simulink model "AM_Multiple_Channels"  (R2014b)
settings: Solver=ode3  StartTime=0.0  StopTime=6  FixedStep=1/5000000  RelTol=1e-3
undefined symbols (not defined in the file or in its folder): dfilt, fdesignblkfcn, gcbh
libraries: dsparch4 x12, commsynccomp2 x8, simulink x8
settings Model: Creator=Eitima  LastModifiedBy=Eitima
settings DataIOCC: ExternalInput=[t,SigTime]  LimitDataPoints=off  LoadExternalInput=on  TimeSaveName=tOut  OutputSaveName=SigTimeOut

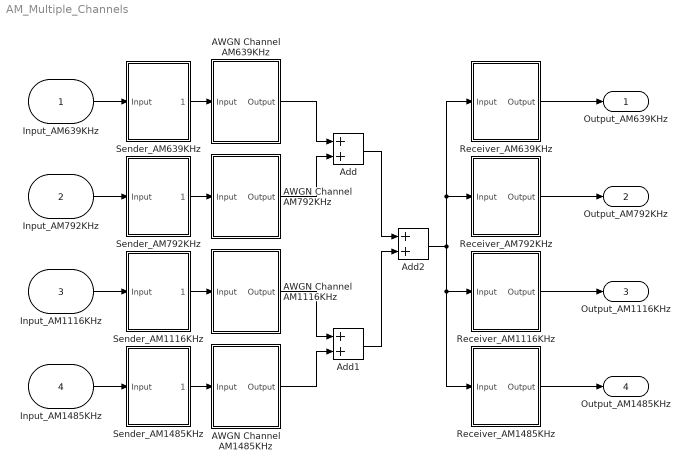
== system AM_Multiple_Channels ==
  Input_AM639KHz : Inport
  Input_AM792KHz : Inport  Port=2
  Input_AM1116KHz : Inport  Port=3
  Input_AM1485KHz : Inport  Port=4
  AWGN Channel AM1116KHz : Subsystem
  AWGN Channel AM1485KHz : Subsystem
  AWGN Channel AM639KHz : Subsystem
  AWGN Channel AM792KHz : Subsystem
  Add : Sum
  Add1 : Sum
  Add2 : Sum
  Receiver_AM1116KHz : Subsystem
  Receiver_AM1485KHz : Subsystem
  Receiver_AM639KHz : Subsystem
  Receiver_AM792KHz : Subsystem
  Sender_AM1116KHz : Subsystem
  Sender_AM1485KHz : Subsystem
  "Sender_AM639KHz " : Subsystem
  Sender_AM792KHz : Subsystem
  Output_AM639KHz : Outport
  Output_AM792KHz : Outport  Port=2
  Output_AM1116KHz : Outport  Port=3
  Output_AM1485KHz : Outport  Port=4
  wires:
  Input_AM639KHz/1 -> "Sender_AM639KHz "/1(Input)
  "Sender_AM639KHz "/1(Output) -> AWGN Channel AM639KHz/1(Input)
  AWGN Channel AM639KHz/1(Output) -> Add/1
  Input_AM792KHz/1 -> Sender_AM792KHz/1(Input)
  Input_AM1116KHz/1 -> Sender_AM1116KHz/1(Input)
  Input_AM1485KHz/1 -> Sender_AM1485KHz/1(Input)
  Sender_AM792KHz/1(Output) -> AWGN Channel AM792KHz/1(Input)
  AWGN Channel AM792KHz/1(Output) -> Add/2
  Sender_AM1116KHz/1(Output) -> AWGN Channel AM1116KHz/1(Input)
  Sender_AM1485KHz/1(Output) -> AWGN Channel AM1485KHz/1(Input)
  AWGN Channel AM1116KHz/1(Output) -> Add1/1
  AWGN Channel AM1485KHz/1(Output) -> Add1/2
  Receiver_AM639KHz/1(Output) -> Output_AM639KHz/1
  Add2/1 -> Receiver_AM1485KHz/1(Input), Receiver_AM1116KHz/1(Input), Receiver_AM792KHz/1(Input), Receiver_AM639KHz/1(Input)
  Add/1 -> Add2/1
  Add1/1 -> Add2/2
  Receiver_AM792KHz/1(Output) -> Output_AM792KHz/1
  Receiver_AM1116KHz/1(Output) -> Output_AM1116KHz/1
  Receiver_AM1485KHz/1(Output) -> Output_AM1485KHz/1

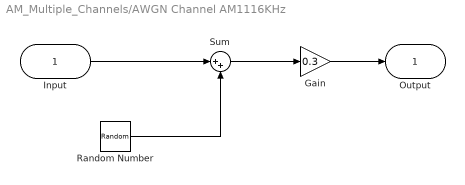
== system AM_Multiple_Channels/AWGN Channel AM1116KHz ==
  Input : Inport
  Gain : Gain  Gain=0.3
  Random Number : RandomNumber  Variance=0.01  Seed=69  SampleTime=1/5000000
  Sum : Sum  Inputs=|++
  Output : Outport
  wires:
  Random Number/1 -> Sum/2
  Input/1 -> Sum/1
  Sum/1 -> Gain/1
  Gain/1 -> Output/1

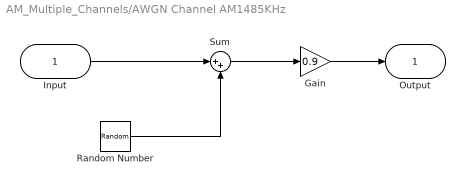
== system AM_Multiple_Channels/AWGN Channel AM1485KHz ==
  Input : Inport
  Gain : Gain  Gain=0.9
  Random Number : RandomNumber  Variance=0.01  Seed=70  SampleTime=1/5000000
  Sum : Sum  Inputs=|++
  Output : Outport
  wires:
  Random Number/1 -> Sum/2
  Input/1 -> Sum/1
  Sum/1 -> Gain/1
  Gain/1 -> Output/1

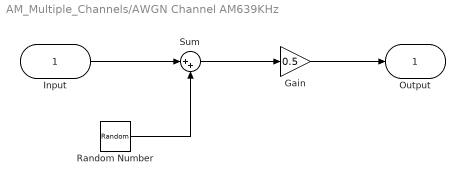
== system AM_Multiple_Channels/AWGN Channel AM639KHz ==
  Input : Inport
  Gain : Gain  Gain=0.5
  Random Number : RandomNumber  Variance=0.01  Seed=64  SampleTime=1/5000000
  Sum : Sum  Inputs=|++
  Output : Outport
  wires:
  Random Number/1 -> Sum/2
  Input/1 -> Sum/1
  Sum/1 -> Gain/1
  Gain/1 -> Output/1

== system AM_Multiple_Channels/AWGN Channel AM792KHz ==
  Input : Inport
  Gain : Gain
  Random Number : RandomNumber  Variance=0.01  Seed=67  SampleTime=1/5000000
  Sum : Sum  Inputs=|++
  Output : Outport
  wires:
  Random Number/1 -> Sum/2
  Input/1 -> Sum/1
  Sum/1 -> Gain/1
  Gain/1 -> Output/1

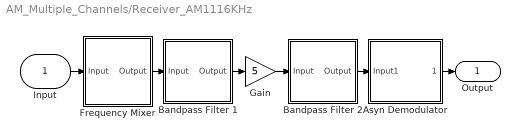
== system AM_Multiple_Channels/Receiver_AM1116KHz ==
  Input : Inport
  Asyn Demodulator : Subsystem
  Bandpass Filter 1 : Subsystem
  Bandpass Filter 2 : Subsystem
  "Frequency Mixer " : Subsystem
  Gain : Gain  Gain=5
  Output : Outport
  wires:
  Input/1 -> "Frequency Mixer "/1(Input)
  "Frequency Mixer "/1(Output) -> Bandpass Filter 1/1(Input)
  Bandpass Filter 1/1(Output) -> Gain/1
  Gain/1 -> Bandpass Filter 2/1(Input)
  Bandpass Filter 2/1(Output) -> Asyn Demodulator/1(Input1)
  Asyn Demodulator/1(Output1) -> Output/1

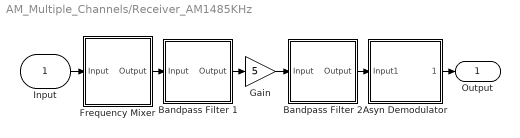
== system AM_Multiple_Channels/Receiver_AM1485KHz ==
  Input : Inport
  Asyn Demodulator : Subsystem
  Bandpass Filter 1 : Subsystem
  Bandpass Filter 2 : Subsystem
  "Frequency Mixer " : Subsystem
  Gain : Gain  Gain=5
  Output : Outport
  wires:
  Input/1 -> "Frequency Mixer "/1(Input)
  "Frequency Mixer "/1(Output) -> Bandpass Filter 1/1(Input)
  Bandpass Filter 1/1(Output) -> Gain/1
  Gain/1 -> Bandpass Filter 2/1(Input)
  Bandpass Filter 2/1(Output) -> Asyn Demodulator/1(Input1)
  Asyn Demodulator/1(Output1) -> Output/1

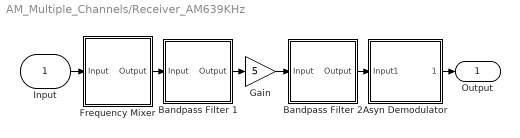
== system AM_Multiple_Channels/Receiver_AM639KHz ==
  Input : Inport
  Asyn Demodulator : Subsystem
  Bandpass Filter 1 : Subsystem
  Bandpass Filter 2 : Subsystem
  "Frequency Mixer " : Subsystem
  Gain : Gain  Gain=5
  Output : Outport
  wires:
  Input/1 -> "Frequency Mixer "/1(Input)
  "Frequency Mixer "/1(Output) -> Bandpass Filter 1/1(Input)
  Bandpass Filter 1/1(Output) -> Gain/1
  Gain/1 -> Bandpass Filter 2/1(Input)
  Bandpass Filter 2/1(Output) -> Asyn Demodulator/1(Input1)
  Asyn Demodulator/1(Output1) -> Output/1

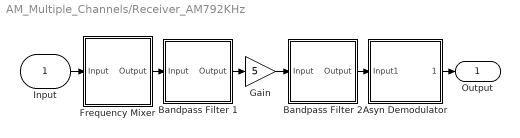
== system AM_Multiple_Channels/Receiver_AM792KHz ==
  Input : Inport
  Asyn Demodulator : Subsystem
  Bandpass Filter 1 : Subsystem
  Bandpass Filter 2 : Subsystem
  "Frequency Mixer " : Subsystem
  Gain : Gain  Gain=5
  Output : Outport
  wires:
  Input/1 -> "Frequency Mixer "/1(Input)
  "Frequency Mixer "/1(Output) -> Bandpass Filter 1/1(Input)
  Bandpass Filter 1/1(Output) -> Gain/1
  Gain/1 -> Bandpass Filter 2/1(Input)
  Bandpass Filter 2/1(Output) -> Asyn Demodulator/1(Input1)
  Asyn Demodulator/1(Output1) -> Output/1

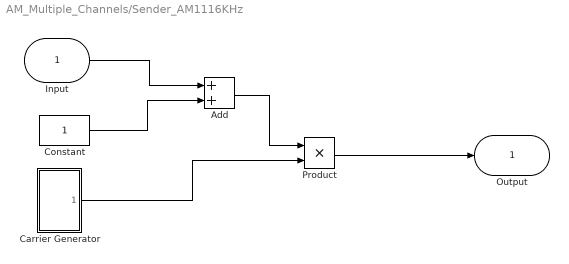
== system AM_Multiple_Channels/Sender_AM1116KHz ==
  Input : Inport
  Add : Sum
  Carrier Generator : Subsystem
  Constant : Constant
  Product : Product
  Output : Outport
  wires:
  Input/1 -> Add/1
  Constant/1 -> Add/2
  Product/1 -> Output/1
  Add/1 -> Product/1
  Carrier Generator/1(Carrier) -> Product/2

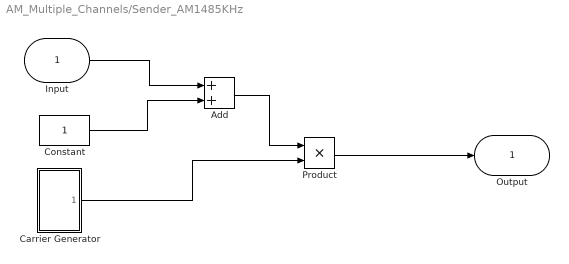
== system AM_Multiple_Channels/Sender_AM1485KHz ==
  Input : Inport
  Add : Sum
  Carrier Generator : Subsystem
  Constant : Constant
  Product : Product
  Output : Outport
  wires:
  Input/1 -> Add/1
  Constant/1 -> Add/2
  Product/1 -> Output/1
  Add/1 -> Product/1
  Carrier Generator/1(Carrier) -> Product/2

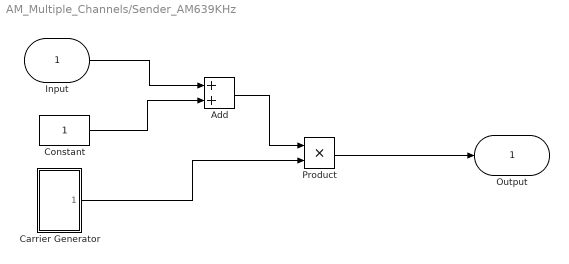
== system AM_Multiple_Channels/Sender_AM639KHz  ==
  Input : Inport
  Add : Sum
  Carrier Generator : Subsystem
  Constant : Constant
  Product : Product
  Output : Outport
  wires:
  Input/1 -> Add/1
  Constant/1 -> Add/2
  Product/1 -> Output/1
  Add/1 -> Product/1
  Carrier Generator/1(Carrier) -> Product/2

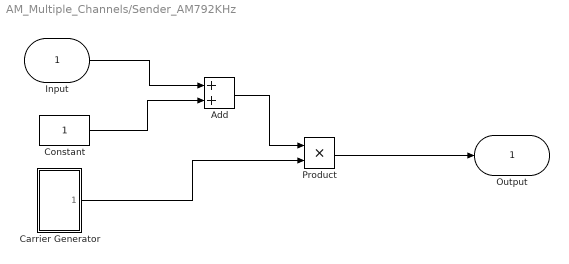
== system AM_Multiple_Channels/Sender_AM792KHz ==
  Input : Inport
  Add : Sum
  Carrier Generator : Subsystem
  Constant : Constant
  Product : Product
  Output : Outport
  wires:
  Input/1 -> Add/1
  Constant/1 -> Add/2
  Product/1 -> Output/1
  Add/1 -> Product/1
  Carrier Generator/1(Carrier) -> Product/2

== system AM_Multiple_Channels/Receiver_AM1116KHz/Asyn Demodulator ==
  Input1 : Inport
  Lowpass Filter1 : Subsystem
  Saturation : Saturate  UpperLimit=inf  LowerLimit=0
  Output1 : Outport
  wires:
  Lowpass Filter1/1(Output) -> Output1/1
  Saturation/1 -> Lowpass Filter1/1(Input)
  Input1/1 -> Saturation/1

== system AM_Multiple_Channels/Receiver_AM1116KHz/Bandpass Filter 1 ==
  Input : Inport
  Bandpass Filter1 : Subsystem  DialogController=fdesignblkfcn  InitFcn=fdesignblkfcn(gcbh, {'InitFcn'});  mask(Bandpass Filter){}
      mask help: Design a bandpass filter
      settings: CopyFcn=fdesignblkfcn(gcbh, {'CopyFcn'});
      mask Help: helpview(mapfilelocation('dsp'), 'dspbandpassfilter');
      mask Display: disp('Bandpass');
  Reshape1 : Reshape
  Zero-Order Hold : ZeroOrderHold  SampleTime=-1
  Output : Outport
  wires:
  Zero-Order Hold/1 -> Bandpass Filter1/1(In)
  Input/1 -> Zero-Order Hold/1
  Bandpass Filter1/1(Out) -> Reshape1/1
  Reshape1/1 -> Output/1

== system AM_Multiple_Channels/Receiver_AM1116KHz/Bandpass Filter 2 ==
  Input : Inport
  Bandpass Filter1 : Subsystem  DialogController=fdesignblkfcn  InitFcn=fdesignblkfcn(gcbh, {'InitFcn'});  mask(Bandpass Filter){}
      mask help: Design a bandpass filter
      settings: CopyFcn=fdesignblkfcn(gcbh, {'CopyFcn'});
      mask Help: helpview(mapfilelocation('dsp'), 'dspbandpassfilter');
      mask Display: disp('Bandpass');
  Reshape1 : Reshape
  Zero-Order Hold1 : ZeroOrderHold  SampleTime=-1
  Output : Outport
  wires:
  Zero-Order Hold1/1 -> Bandpass Filter1/1(In)
  Input/1 -> Zero-Order Hold1/1
  Bandpass Filter1/1(Out) -> Reshape1/1
  Reshape1/1 -> Output/1

== system AM_Multiple_Channels/Receiver_AM1116KHz/Frequency Mixer  ==
  Input : Inport
  Local Oscilator Signal : Subsystem
  Product : Product
  Output : Outport
  wires:
  Product/1 -> Output/1
  Local Oscilator Signal/1(Output) -> Product/2
  Input/1 -> Product/1

== system AM_Multiple_Channels/Receiver_AM1485KHz/Asyn Demodulator ==
  Input1 : Inport
  Lowpass Filter1 : Subsystem
  Saturation : Saturate  UpperLimit=inf  LowerLimit=0
  Output1 : Outport
  wires:
  Lowpass Filter1/1(Output) -> Output1/1
  Saturation/1 -> Lowpass Filter1/1(Input)
  Input1/1 -> Saturation/1

== system AM_Multiple_Channels/Receiver_AM1485KHz/Bandpass Filter 1 ==
  Input : Inport
  Bandpass Filter1 : Subsystem  DialogController=fdesignblkfcn  InitFcn=fdesignblkfcn(gcbh, {'InitFcn'});  mask(Bandpass Filter){}
      mask help: Design a bandpass filter
      settings: CopyFcn=fdesignblkfcn(gcbh, {'CopyFcn'});
      mask Help: helpview(mapfilelocation('dsp'), 'dspbandpassfilter');
      mask Display: disp('Bandpass');
  Reshape1 : Reshape
  Zero-Order Hold : ZeroOrderHold  SampleTime=-1
  Output : Outport
  wires:
  Zero-Order Hold/1 -> Bandpass Filter1/1(In)
  Input/1 -> Zero-Order Hold/1
  Bandpass Filter1/1(Out) -> Reshape1/1
  Reshape1/1 -> Output/1

== system AM_Multiple_Channels/Receiver_AM1485KHz/Bandpass Filter 2 ==
  Input : Inport
  Bandpass Filter1 : Subsystem  DialogController=fdesignblkfcn  InitFcn=fdesignblkfcn(gcbh, {'InitFcn'});  mask(Bandpass Filter){}
      mask help: Design a bandpass filter
      settings: CopyFcn=fdesignblkfcn(gcbh, {'CopyFcn'});
      mask Help: helpview(mapfilelocation('dsp'), 'dspbandpassfilter');
      mask Display: disp('Bandpass');
  Reshape1 : Reshape
  Zero-Order Hold1 : ZeroOrderHold  SampleTime=-1
  Output : Outport
  wires:
  Zero-Order Hold1/1 -> Bandpass Filter1/1(In)
  Input/1 -> Zero-Order Hold1/1
  Bandpass Filter1/1(Out) -> Reshape1/1
  Reshape1/1 -> Output/1

== system AM_Multiple_Channels/Receiver_AM1485KHz/Frequency Mixer  ==
  Input : Inport
  Local Oscilator Signal : Subsystem
  Product : Product
  Output : Outport
  wires:
  Product/1 -> Output/1
  Local Oscilator Signal/1(Output) -> Product/2
  Input/1 -> Product/1

== system AM_Multiple_Channels/Receiver_AM639KHz/Asyn Demodulator ==
  Input1 : Inport
  Lowpass Filter1 : Subsystem
  Saturation : Saturate  UpperLimit=inf  LowerLimit=0
  Output1 : Outport
  wires:
  Lowpass Filter1/1(Output) -> Output1/1
  Saturation/1 -> Lowpass Filter1/1(Input)
  Input1/1 -> Saturation/1

== system AM_Multiple_Channels/Receiver_AM639KHz/Bandpass Filter 1 ==
  Input : Inport
  Bandpass Filter1 : Subsystem  DialogController=fdesignblkfcn  InitFcn=fdesignblkfcn(gcbh, {'InitFcn'});  mask(Bandpass Filter){}
      mask help: Design a bandpass filter
      settings: CopyFcn=fdesignblkfcn(gcbh, {'CopyFcn'});
      mask Help: helpview(mapfilelocation('dsp'), 'dspbandpassfilter');
      mask Display: disp('Bandpass');
  Reshape1 : Reshape
  Zero-Order Hold : ZeroOrderHold  SampleTime=-1
  Output : Outport
  wires:
  Zero-Order Hold/1 -> Bandpass Filter1/1(In)
  Input/1 -> Zero-Order Hold/1
  Bandpass Filter1/1(Out) -> Reshape1/1
  Reshape1/1 -> Output/1

== system AM_Multiple_Channels/Receiver_AM639KHz/Bandpass Filter 2 ==
  Input : Inport
  Bandpass Filter1 : Subsystem  DialogController=fdesignblkfcn  InitFcn=fdesignblkfcn(gcbh, {'InitFcn'});  mask(Bandpass Filter){}
      mask help: Design a bandpass filter
      settings: CopyFcn=fdesignblkfcn(gcbh, {'CopyFcn'});
      mask Help: helpview(mapfilelocation('dsp'), 'dspbandpassfilter');
      mask Display: disp('Bandpass');
  Reshape1 : Reshape
  Zero-Order Hold1 : ZeroOrderHold  SampleTime=-1
  Output : Outport
  wires:
  Zero-Order Hold1/1 -> Bandpass Filter1/1(In)
  Input/1 -> Zero-Order Hold1/1
  Bandpass Filter1/1(Out) -> Reshape1/1
  Reshape1/1 -> Output/1

== system AM_Multiple_Channels/Receiver_AM639KHz/Frequency Mixer  ==
  Input : Inport
  Local Oscilator Signal : Subsystem
  Product : Product
  Output : Outport
  wires:
  Product/1 -> Output/1
  Local Oscilator Signal/1(Output) -> Product/2
  Input/1 -> Product/1

== system AM_Multiple_Channels/Receiver_AM792KHz/Asyn Demodulator ==
  Input1 : Inport
  Lowpass Filter1 : Subsystem
  Saturation : Saturate  UpperLimit=inf  LowerLimit=0
  Output1 : Outport
  wires:
  Lowpass Filter1/1(Output) -> Output1/1
  Saturation/1 -> Lowpass Filter1/1(Input)
  Input1/1 -> Saturation/1

== system AM_Multiple_Channels/Receiver_AM792KHz/Bandpass Filter 1 ==
  Input : Inport
  Bandpass Filter1 : Subsystem  DialogController=fdesignblkfcn  InitFcn=fdesignblkfcn(gcbh, {'InitFcn'});  mask(Bandpass Filter){}
      mask help: Design a bandpass filter
      settings: CopyFcn=fdesignblkfcn(gcbh, {'CopyFcn'});
      mask Help: helpview(mapfilelocation('dsp'), 'dspbandpassfilter');
      mask Display: disp('Bandpass');
  Reshape1 : Reshape
  Zero-Order Hold : ZeroOrderHold  SampleTime=-1
  Output : Outport
  wires:
  Zero-Order Hold/1 -> Bandpass Filter1/1(In)
  Input/1 -> Zero-Order Hold/1
  Bandpass Filter1/1(Out) -> Reshape1/1
  Reshape1/1 -> Output/1

== system AM_Multiple_Channels/Receiver_AM792KHz/Bandpass Filter 2 ==
  Input : Inport
  Bandpass Filter1 : Subsystem  DialogController=fdesignblkfcn  InitFcn=fdesignblkfcn(gcbh, {'InitFcn'});  mask(Bandpass Filter){}
      mask help: Design a bandpass filter
      settings: CopyFcn=fdesignblkfcn(gcbh, {'CopyFcn'});
      mask Help: helpview(mapfilelocation('dsp'), 'dspbandpassfilter');
      mask Display: disp('Bandpass');
  Reshape1 : Reshape
  Zero-Order Hold1 : ZeroOrderHold  SampleTime=-1
  Output : Outport
  wires:
  Zero-Order Hold1/1 -> Bandpass Filter1/1(In)
  Input/1 -> Zero-Order Hold1/1
  Bandpass Filter1/1(Out) -> Reshape1/1
  Reshape1/1 -> Output/1

== system AM_Multiple_Channels/Receiver_AM792KHz/Frequency Mixer  ==
  Input : Inport
  Local Oscilator Signal : Subsystem
  Product : Product
  Output : Outport
  wires:
  Product/1 -> Output/1
  Local Oscilator Signal/1(Output) -> Product/2
  Input/1 -> Product/1

== system AM_Multiple_Channels/Sender_AM1116KHz/Carrier Generator ==
  Constant1 : Constant
  Discrete-Time VCO : commsynccomp2/Discrete-Time VCO  Ac=1  Fc=0  Kc=1000  Ph=0  ts=1/5000000
  Slider Gain : simulink/Math Operations/Slider Gain  low=550  gain=1116  high=1605
  Carrier : Outport
  wires:
  Discrete-Time VCO/1 -> Carrier/1
  Slider Gain/1 -> Discrete-Time VCO/1
  Constant1/1 -> Slider Gain/1

== system AM_Multiple_Channels/Sender_AM1485KHz/Carrier Generator ==
  Constant1 : Constant
  Discrete-Time VCO : commsynccomp2/Discrete-Time VCO  Ac=1  Fc=0  Kc=1000  Ph=0  ts=1/5000000
  Slider Gain : simulink/Math Operations/Slider Gain  low=550  gain=1485  high=1605
  Carrier : Outport
  wires:
  Discrete-Time VCO/1 -> Carrier/1
  Slider Gain/1 -> Discrete-Time VCO/1
  Constant1/1 -> Slider Gain/1

== system AM_Multiple_Channels/Sender_AM639KHz /Carrier Generator ==
  Constant1 : Constant
  Discrete-Time VCO : commsynccomp2/Discrete-Time VCO  Ac=1  Fc=0  Kc=1000  Ph=0  ts=1/5000000
  Slider Gain : simulink/Math Operations/Slider Gain  low=550  gain=639  high=1605
  Carrier : Outport
  wires:
  Discrete-Time VCO/1 -> Carrier/1
  Slider Gain/1 -> Discrete-Time VCO/1
  Constant1/1 -> Slider Gain/1

== system AM_Multiple_Channels/Sender_AM792KHz/Carrier Generator ==
  Constant1 : Constant
  Discrete-Time VCO : commsynccomp2/Discrete-Time VCO  Ac=1  Fc=0  Kc=1000  Ph=0  ts=1/5000000
  Slider Gain : simulink/Math Operations/Slider Gain  low=550  gain=792  high=1605
  Carrier : Outport
  wires:
  Discrete-Time VCO/1 -> Carrier/1
  Slider Gain/1 -> Discrete-Time VCO/1
  Constant1/1 -> Slider Gain/1

== system AM_Multiple_Channels/Receiver_AM1116KHz/Asyn Demodulator/Lowpass Filter1 ==
  Input : Inport
  Lowpass Filter : Subsystem  DialogController=fdesignblkfcn  InitFcn=fdesignblkfcn(gcbh, {'InitFcn'});  mask(Lowpass Filter){}
      mask help: Design a lowpass filter
      settings: CopyFcn=fdesignblkfcn(gcbh, {'CopyFcn'});
      mask Help: helpview(mapfilelocation('dsp'), 'dsplowpassfilter');
      mask Display: disp('Lowpass')
  Reshape : Reshape
  Zero-Order Hold1 : ZeroOrderHold  SampleTime=-1
  Output : Outport
  wires:
  Zero-Order Hold1/1 -> Lowpass Filter/1(In)
  Input/1 -> Zero-Order Hold1/1
  Lowpass Filter/1(Out) -> Reshape/1
  Reshape/1 -> Output/1

== system AM_Multiple_Channels/Receiver_AM1116KHz/Bandpass Filter 1/Bandpass Filter1 ==
  In : Inport
  Generated Filter Block : dsparch4/Biquad Filter  Tag=BlockMethodSubSystem  IIRFiltStruct=Direct form II  CoeffSource=Specify via dialog  BiQuadCoeffs=[0.01013958648634297 0 -0.01013958648634297 1 -1.6618133812024951 0.98627046054740486;0.0025493781187891492 0 -0.0025493781187891492 1 -1.6514591991218408 0.98607730419032968;0.016304485317952876 0 -0.016304485317952876 1 -1.6744504392878072 0.99677925049276372;0.010019474414157988 0 -0.010019474414157988 1 -1.6562936076737262 0.99669840495107032;0.011567698875754661 0 -0.011567698875754661 1 -1.6564338939134684 0.98375080085450683;0.0047790385123797378 0 -0.0047790385123797378 1 -1.6527923586273903 0.98367098468879577;0.014421092390225715 0 -0.014421092390225715 1 -1.6681267322604891 0.99083770350510236;0.91340939446196634 0 -0.91340939446196634 1 -1.6526752268318703 0.99064368018868598]  a0Flag=Warning  IC=0  ICnum=0  ICden=0  InputProcessing=Columns as channels (frame based)  denAccumFracLength=30  denProdOutputFracLength=30  secondMemoryFracLength=15  roundingMode=Floor  overflowMode=off  ScaleValues=[0.0075209697231768506;1;1;1;1;1;1;1;1]  optimizeScaleValues=off  ScaleValueMode=Specify via input port (g)  scaleValueFracLength=14  FilterSource=Specify via dialog  dfiltObjectName=dfilt.df2tsos([1 0.3 0.4],[1 0.1 0.2])
  Out : Outport
  wires:
  Generated Filter Block/1 -> Out/1
  In/1 -> Generated Filter Block/1

== system AM_Multiple_Channels/Receiver_AM1116KHz/Bandpass Filter 2/Bandpass Filter1 ==
  In : Inport
  Generated Filter Block : dsparch4/Biquad Filter  Tag=BlockMethodSubSystem  IIRFiltStruct=Direct form II  CoeffSource=Specify via dialog  BiQuadCoeffs=[0.01013958648634297 0 -0.01013958648634297 1 -1.6618133812024951 0.98627046054740486;0.0025493781187891492 0 -0.0025493781187891492 1 -1.6514591991218408 0.98607730419032968;0.016304485317952876 0 -0.016304485317952876 1 -1.6744504392878072 0.99677925049276372;0.010019474414157988 0 -0.010019474414157988 1 -1.6562936076737262 0.99669840495107032;0.011567698875754661 0 -0.011567698875754661 1 -1.6564338939134684 0.98375080085450683;0.0047790385123797378 0 -0.0047790385123797378 1 -1.6527923586273903 0.98367098468879577;0.014421092390225715 0 -0.014421092390225715 1 -1.6681267322604891 0.99083770350510236;0.91340939446196634 0 -0.91340939446196634 1 -1.6526752268318703 0.99064368018868598]  a0Flag=Warning  IC=0  ICnum=0  ICden=0  InputProcessing=Columns as channels (frame based)  denAccumFracLength=30  denProdOutputFracLength=30  secondMemoryFracLength=15  roundingMode=Floor  overflowMode=off  ScaleValues=[0.0075209697231768506;1;1;1;1;1;1;1;1]  optimizeScaleValues=off  ScaleValueMode=Specify via input port (g)  scaleValueFracLength=14  FilterSource=Specify via dialog  dfiltObjectName=dfilt.df2tsos([1 0.3 0.4],[1 0.1 0.2])
  Out : Outport
  wires:
  Generated Filter Block/1 -> Out/1
  In/1 -> Generated Filter Block/1

== system AM_Multiple_Channels/Receiver_AM1116KHz/Frequency Mixer /Local Oscilator Signal ==
  Constant : Constant
  Discrete-Time VCO : commsynccomp2/Discrete-Time VCO  Ac=1  Fc=0  Kc=1000  Ph=0  ts=1/5000000
  Slider Gain : simulink/Math Operations/Slider Gain  low=1015  gain=1581  high=2070
  Output : Outport
  wires:
  Discrete-Time VCO/1 -> Output/1
  Slider Gain/1 -> Discrete-Time VCO/1
  Constant/1 -> Slider Gain/1

== system AM_Multiple_Channels/Receiver_AM1485KHz/Asyn Demodulator/Lowpass Filter1 ==
  Input : Inport
  Lowpass Filter : Subsystem  DialogController=fdesignblkfcn  InitFcn=fdesignblkfcn(gcbh, {'InitFcn'});  mask(Lowpass Filter){}
      mask help: Design a lowpass filter
      settings: CopyFcn=fdesignblkfcn(gcbh, {'CopyFcn'});
      mask Help: helpview(mapfilelocation('dsp'), 'dsplowpassfilter');
      mask Display: disp('Lowpass')
  Reshape : Reshape
  Zero-Order Hold1 : ZeroOrderHold  SampleTime=-1
  Output : Outport
  wires:
  Zero-Order Hold1/1 -> Lowpass Filter/1(In)
  Input/1 -> Zero-Order Hold1/1
  Lowpass Filter/1(Out) -> Reshape/1
  Reshape/1 -> Output/1

== system AM_Multiple_Channels/Receiver_AM1485KHz/Bandpass Filter 1/Bandpass Filter1 ==
  In : Inport
  Generated Filter Block : dsparch4/Biquad Filter  Tag=BlockMethodSubSystem  IIRFiltStruct=Direct form II  CoeffSource=Specify via dialog  BiQuadCoeffs=[0.01013958648634297 0 -0.01013958648634297 1 -1.6618133812024951 0.98627046054740486;0.0025493781187891492 0 -0.0025493781187891492 1 -1.6514591991218408 0.98607730419032968;0.016304485317952876 0 -0.016304485317952876 1 -1.6744504392878072 0.99677925049276372;0.010019474414157988 0 -0.010019474414157988 1 -1.6562936076737262 0.99669840495107032;0.011567698875754661 0 -0.011567698875754661 1 -1.6564338939134684 0.98375080085450683;0.0047790385123797378 0 -0.0047790385123797378 1 -1.6527923586273903 0.98367098468879577;0.014421092390225715 0 -0.014421092390225715 1 -1.6681267322604891 0.99083770350510236;0.91340939446196634 0 -0.91340939446196634 1 -1.6526752268318703 0.99064368018868598]  a0Flag=Warning  IC=0  ICnum=0  ICden=0  InputProcessing=Columns as channels (frame based)  denAccumFracLength=30  denProdOutputFracLength=30  secondMemoryFracLength=15  roundingMode=Floor  overflowMode=off  ScaleValues=[0.0075209697231768506;1;1;1;1;1;1;1;1]  optimizeScaleValues=off  ScaleValueMode=Specify via input port (g)  scaleValueFracLength=14  FilterSource=Specify via dialog  dfiltObjectName=dfilt.df2tsos([1 0.3 0.4],[1 0.1 0.2])
  Out : Outport
  wires:
  Generated Filter Block/1 -> Out/1
  In/1 -> Generated Filter Block/1

== system AM_Multiple_Channels/Receiver_AM1485KHz/Bandpass Filter 2/Bandpass Filter1 ==
  In : Inport
  Generated Filter Block : dsparch4/Biquad Filter  Tag=BlockMethodSubSystem  IIRFiltStruct=Direct form II  CoeffSource=Specify via dialog  BiQuadCoeffs=[0.01013958648634297 0 -0.01013958648634297 1 -1.6618133812024951 0.98627046054740486;0.0025493781187891492 0 -0.0025493781187891492 1 -1.6514591991218408 0.98607730419032968;0.016304485317952876 0 -0.016304485317952876 1 -1.6744504392878072 0.99677925049276372;0.010019474414157988 0 -0.010019474414157988 1 -1.6562936076737262 0.99669840495107032;0.011567698875754661 0 -0.011567698875754661 1 -1.6564338939134684 0.98375080085450683;0.0047790385123797378 0 -0.0047790385123797378 1 -1.6527923586273903 0.98367098468879577;0.014421092390225715 0 -0.014421092390225715 1 -1.6681267322604891 0.99083770350510236;0.91340939446196634 0 -0.91340939446196634 1 -1.6526752268318703 0.99064368018868598]  a0Flag=Warning  IC=0  ICnum=0  ICden=0  InputProcessing=Columns as channels (frame based)  denAccumFracLength=30  denProdOutputFracLength=30  secondMemoryFracLength=15  roundingMode=Floor  overflowMode=off  ScaleValues=[0.0075209697231768506;1;1;1;1;1;1;1;1]  optimizeScaleValues=off  ScaleValueMode=Specify via input port (g)  scaleValueFracLength=14  FilterSource=Specify via dialog  dfiltObjectName=dfilt.df2tsos([1 0.3 0.4],[1 0.1 0.2])
  Out : Outport
  wires:
  Generated Filter Block/1 -> Out/1
  In/1 -> Generated Filter Block/1

== system AM_Multiple_Channels/Receiver_AM1485KHz/Frequency Mixer /Local Oscilator Signal ==
  Constant : Constant
  Discrete-Time VCO : commsynccomp2/Discrete-Time VCO  Ac=1  Fc=0  Kc=1000  Ph=0  ts=1/5000000
  Slider Gain : simulink/Math Operations/Slider Gain  low=1015  gain=1950  high=2070
  Output : Outport
  wires:
  Discrete-Time VCO/1 -> Output/1
  Slider Gain/1 -> Discrete-Time VCO/1
  Constant/1 -> Slider Gain/1

== system AM_Multiple_Channels/Receiver_AM639KHz/Asyn Demodulator/Lowpass Filter1 ==
  Input : Inport
  Lowpass Filter : Subsystem  DialogController=fdesignblkfcn  InitFcn=fdesignblkfcn(gcbh, {'InitFcn'});  mask(Lowpass Filter){}
      mask help: Design a lowpass filter
      settings: CopyFcn=fdesignblkfcn(gcbh, {'CopyFcn'});
      mask Help: helpview(mapfilelocation('dsp'), 'dsplowpassfilter');
      mask Display: disp('Lowpass')
  Reshape : Reshape
  Zero-Order Hold1 : ZeroOrderHold  SampleTime=-1
  Output : Outport
  wires:
  Zero-Order Hold1/1 -> Lowpass Filter/1(In)
  Input/1 -> Zero-Order Hold1/1
  Lowpass Filter/1(Out) -> Reshape/1
  Reshape/1 -> Output/1

== system AM_Multiple_Channels/Receiver_AM639KHz/Bandpass Filter 1/Bandpass Filter1 ==
  In : Inport
  Generated Filter Block : dsparch4/Biquad Filter  Tag=BlockMethodSubSystem  IIRFiltStruct=Direct form II  CoeffSource=Specify via dialog  BiQuadCoeffs=[0.01013958648634297 0 -0.01013958648634297 1 -1.6618133812024951 0.98627046054740486;0.0025493781187891492 0 -0.0025493781187891492 1 -1.6514591991218408 0.98607730419032968;0.016304485317952876 0 -0.016304485317952876 1 -1.6744504392878072 0.99677925049276372;0.010019474414157988 0 -0.010019474414157988 1 -1.6562936076737262 0.99669840495107032;0.011567698875754661 0 -0.011567698875754661 1 -1.6564338939134684 0.98375080085450683;0.0047790385123797378 0 -0.0047790385123797378 1 -1.6527923586273903 0.98367098468879577;0.014421092390225715 0 -0.014421092390225715 1 -1.6681267322604891 0.99083770350510236;0.91340939446196634 0 -0.91340939446196634 1 -1.6526752268318703 0.99064368018868598]  a0Flag=Warning  IC=0  ICnum=0  ICden=0  InputProcessing=Columns as channels (frame based)  denAccumFracLength=30  denProdOutputFracLength=30  secondMemoryFracLength=15  roundingMode=Floor  overflowMode=off  ScaleValues=[0.0075209697231768506;1;1;1;1;1;1;1;1]  optimizeScaleValues=off  ScaleValueMode=Specify via input port (g)  scaleValueFracLength=14  FilterSource=Specify via dialog  dfiltObjectName=dfilt.df2tsos([1 0.3 0.4],[1 0.1 0.2])
  Out : Outport
  wires:
  Generated Filter Block/1 -> Out/1
  In/1 -> Generated Filter Block/1

== system AM_Multiple_Channels/Receiver_AM639KHz/Bandpass Filter 2/Bandpass Filter1 ==
  In : Inport
  Generated Filter Block : dsparch4/Biquad Filter  Tag=BlockMethodSubSystem  IIRFiltStruct=Direct form II  CoeffSource=Specify via dialog  BiQuadCoeffs=[0.01013958648634297 0 -0.01013958648634297 1 -1.6618133812024951 0.98627046054740486;0.0025493781187891492 0 -0.0025493781187891492 1 -1.6514591991218408 0.98607730419032968;0.016304485317952876 0 -0.016304485317952876 1 -1.6744504392878072 0.99677925049276372;0.010019474414157988 0 -0.010019474414157988 1 -1.6562936076737262 0.99669840495107032;0.011567698875754661 0 -0.011567698875754661 1 -1.6564338939134684 0.98375080085450683;0.0047790385123797378 0 -0.0047790385123797378 1 -1.6527923586273903 0.98367098468879577;0.014421092390225715 0 -0.014421092390225715 1 -1.6681267322604891 0.99083770350510236;0.91340939446196634 0 -0.91340939446196634 1 -1.6526752268318703 0.99064368018868598]  a0Flag=Warning  IC=0  ICnum=0  ICden=0  InputProcessing=Columns as channels (frame based)  denAccumFracLength=30  denProdOutputFracLength=30  secondMemoryFracLength=15  roundingMode=Floor  overflowMode=off  ScaleValues=[0.0075209697231768506;1;1;1;1;1;1;1;1]  optimizeScaleValues=off  ScaleValueMode=Specify via input port (g)  scaleValueFracLength=14  FilterSource=Specify via dialog  dfiltObjectName=dfilt.df2tsos([1 0.3 0.4],[1 0.1 0.2])
  Out : Outport
  wires:
  Generated Filter Block/1 -> Out/1
  In/1 -> Generated Filter Block/1

== system AM_Multiple_Channels/Receiver_AM639KHz/Frequency Mixer /Local Oscilator Signal ==
  Constant : Constant
  Discrete-Time VCO : commsynccomp2/Discrete-Time VCO  Ac=1  Fc=0  Kc=1000  Ph=0  ts=1/5000000
  Slider Gain : simulink/Math Operations/Slider Gain  low=1015  gain=1104  high=2070
  Output : Outport
  wires:
  Discrete-Time VCO/1 -> Output/1
  Slider Gain/1 -> Discrete-Time VCO/1
  Constant/1 -> Slider Gain/1

== system AM_Multiple_Channels/Receiver_AM792KHz/Asyn Demodulator/Lowpass Filter1 ==
  Input : Inport
  Lowpass Filter : Subsystem  DialogController=fdesignblkfcn  InitFcn=fdesignblkfcn(gcbh, {'InitFcn'});  mask(Lowpass Filter){}
      mask help: Design a lowpass filter
      settings: CopyFcn=fdesignblkfcn(gcbh, {'CopyFcn'});
      mask Help: helpview(mapfilelocation('dsp'), 'dsplowpassfilter');
      mask Display: disp('Lowpass')
  Reshape : Reshape
  Zero-Order Hold1 : ZeroOrderHold  SampleTime=-1
  Output : Outport
  wires:
  Zero-Order Hold1/1 -> Lowpass Filter/1(In)
  Input/1 -> Zero-Order Hold1/1
  Lowpass Filter/1(Out) -> Reshape/1
  Reshape/1 -> Output/1

== system AM_Multiple_Channels/Receiver_AM792KHz/Bandpass Filter 1/Bandpass Filter1 ==
  In : Inport
  Generated Filter Block : dsparch4/Biquad Filter  Tag=BlockMethodSubSystem  IIRFiltStruct=Direct form II  CoeffSource=Specify via dialog  BiQuadCoeffs=[0.01013958648634297 0 -0.01013958648634297 1 -1.6618133812024951 0.98627046054740486;0.0025493781187891492 0 -0.0025493781187891492 1 -1.6514591991218408 0.98607730419032968;0.016304485317952876 0 -0.016304485317952876 1 -1.6744504392878072 0.99677925049276372;0.010019474414157988 0 -0.010019474414157988 1 -1.6562936076737262 0.99669840495107032;0.011567698875754661 0 -0.011567698875754661 1 -1.6564338939134684 0.98375080085450683;0.0047790385123797378 0 -0.0047790385123797378 1 -1.6527923586273903 0.98367098468879577;0.014421092390225715 0 -0.014421092390225715 1 -1.6681267322604891 0.99083770350510236;0.91340939446196634 0 -0.91340939446196634 1 -1.6526752268318703 0.99064368018868598]  a0Flag=Warning  IC=0  ICnum=0  ICden=0  InputProcessing=Columns as channels (frame based)  denAccumFracLength=30  denProdOutputFracLength=30  secondMemoryFracLength=15  roundingMode=Floor  overflowMode=off  ScaleValues=[0.0075209697231768506;1;1;1;1;1;1;1;1]  optimizeScaleValues=off  ScaleValueMode=Specify via input port (g)  scaleValueFracLength=14  FilterSource=Specify via dialog  dfiltObjectName=dfilt.df2tsos([1 0.3 0.4],[1 0.1 0.2])
  Out : Outport
  wires:
  Generated Filter Block/1 -> Out/1
  In/1 -> Generated Filter Block/1

== system AM_Multiple_Channels/Receiver_AM792KHz/Bandpass Filter 2/Bandpass Filter1 ==
  In : Inport
  Generated Filter Block : dsparch4/Biquad Filter  Tag=BlockMethodSubSystem  IIRFiltStruct=Direct form II  CoeffSource=Specify via dialog  BiQuadCoeffs=[0.01013958648634297 0 -0.01013958648634297 1 -1.6618133812024951 0.98627046054740486;0.0025493781187891492 0 -0.0025493781187891492 1 -1.6514591991218408 0.98607730419032968;0.016304485317952876 0 -0.016304485317952876 1 -1.6744504392878072 0.99677925049276372;0.010019474414157988 0 -0.010019474414157988 1 -1.6562936076737262 0.99669840495107032;0.011567698875754661 0 -0.011567698875754661 1 -1.6564338939134684 0.98375080085450683;0.0047790385123797378 0 -0.0047790385123797378 1 -1.6527923586273903 0.98367098468879577;0.014421092390225715 0 -0.014421092390225715 1 -1.6681267322604891 0.99083770350510236;0.91340939446196634 0 -0.91340939446196634 1 -1.6526752268318703 0.99064368018868598]  a0Flag=Warning  IC=0  ICnum=0  ICden=0  InputProcessing=Columns as channels (frame based)  denAccumFracLength=30  denProdOutputFracLength=30  secondMemoryFracLength=15  roundingMode=Floor  overflowMode=off  ScaleValues=[0.0075209697231768506;1;1;1;1;1;1;1;1]  optimizeScaleValues=off  ScaleValueMode=Specify via input port (g)  scaleValueFracLength=14  FilterSource=Specify via dialog  dfiltObjectName=dfilt.df2tsos([1 0.3 0.4],[1 0.1 0.2])
  Out : Outport
  wires:
  Generated Filter Block/1 -> Out/1
  In/1 -> Generated Filter Block/1

== system AM_Multiple_Channels/Receiver_AM792KHz/Frequency Mixer /Local Oscilator Signal ==
  Constant : Constant
  Discrete-Time VCO : commsynccomp2/Discrete-Time VCO  Ac=1  Fc=0  Kc=1000  Ph=0  ts=1/5000000
  Slider Gain : simulink/Math Operations/Slider Gain  low=1015  gain=1257  high=2070
  Output : Outport
  wires:
  Discrete-Time VCO/1 -> Output/1
  Slider Gain/1 -> Discrete-Time VCO/1
  Constant/1 -> Slider Gain/1

== system AM_Multiple_Channels/Receiver_AM1116KHz/Asyn Demodulator/Lowpass Filter1/Lowpass Filter ==
  In : Inport
  Generated Filter Block : dsparch4/Biquad Filter  Tag=BlockMethodSubSystem  IIRFiltStruct=Direct form II  CoeffSource=Specify via dialog  BiQuadCoeffs=[1.1139495474470017e-05 2.2278990948940034e-05 1.1139495474470017e-05 1 -1.9975472496899784 0.99760587630988296;1.708449290031526e-05 3.4168985800630521e-05 1.708449290031526e-05 1 -1.99387457640288 0.99393309523238282;2.1150286544110928e-05 4.2300573088221855e-05 2.1150286544110928e-05 1 -1.9905941002634866 0.99065252281330018;2.3741131754506419e-05 4.7482263509012838e-05 2.3741131754506419e-05 1 -1.9879072271736171 0.9879655708655779;2.2148688266151217e-05 4.4297376532302434e-05 2.2148688266151217e-05 1 -1.9859774513096744 0.98603573836405833;1.4562706238119281e-05 2.9125412476238562e-05 1.4562706238119281e-05 1 -1.9849213847063547 0.98497964076591971;1.4567049256231092e-05 2.9134098512462184e-05 1.4567049256231092e-05 1 -1.9847430291087753 0.98480127993372768;1.457808673549499e-05 2.915617347098998e-05 1.457808673549499e-05 1 -1.9853349366021702 0.98539320479919512;1.4595153426943952e-05 2.9190306853887904e-05 1.4595153426943952e-05 1 -1.986839228435767 0.98689754078270897;1.4617214727563608e-05 2.9234429455127217e-05 1.4617214727563608e-05 1 -1.9891652381977778 0.98922361881148557;1.4642922502972056e-05 2.9285845005944111e-05 1.4642922502972056e-05 1 -1.9921719604380583 0.99223042929696859;8.6714112246987757e-06 1.7342822449397551e-05 8.6714112246987757e-06 1 -1.995675658652956 0.99573423034296782;6.3986527910792821e-06 1.2797305582158564e-05 6.3986527910792821e-06 1 -1.9994601364673172 0.99951881922911578;1.3142520276408514e-05 2.6285040552817028e-05 1.3142520276408514e-05 1 -1.9966044420030755 0.99666304095223146;1.8418289343954956e-05 3.6836578687909913e-05 1.8418289343954956e-05 1 -1.9930092733310447 0.99306776676450537;2.2982277427308612e-05 4.5964554854617224e-05 2.2982277427308612e-05 1 -1.9898596189140614 0.98991801990735939;2.6110938013399351e-05 5.2221876026798703e-05 2.6110938013399351e-05 1 -1.9873483912460574 0.98740671853657336;1.7614429604367743e-05 3.5228859208735487e-05 1.7614429604367743e-05 1 -1.9856280998827738 0.98568637668393688;1.4565318613601885e-05 2.9130637227203771e-05 1.4565318613601885e-05 1 -1.9848025557236171 0.98486080829563394;1.4574729484739814e-05 2.9149458969479628e-05 1.4574729484739814e-05 1 -1.9850990682844676 0.98515732955892188;1.4590372236056304e-05 2.9180744472112607e-05 1.4590372236056304e-05 1 -1.9863816706239454 0.98643996954188451;1.4611300168831942e-05 2.9222600337663884e-05 1.4611300168831942e-05 1 -1.9885136123818619 0.98857197387080598;1.4636237197718225e-05 2.9272474395436451e-05 1.4636237197718225e-05 1 -1.9913658685524318 0.99142431375310713;1.4663493412127055e-05 2.9326986824254111e-05 1.4663493412127055e-05 1 -1.9947645221736521 0.99482306712244295;0.25000264423165819 0.50000528846331638 0.25000264423165819 1 -1.9985003940838757 0.99855904867790413]  a0Flag=Warning  IC=0  ICnum=0  ICden=0  InputProcessing=Columns as channels (frame based)  denAccumFracLength=30  denProdOutputFracLength=30  secondMemoryFracLength=15  roundingMode=Floor  overflowMode=off  ScaleValues=[1.8320818000818615e-05;1;1;1;1;1;1;1;1;1;1;1;1;1;1;1;1;1;1;1;1;1;1;1;1;1]  optimizeScaleValues=off  ScaleValueMode=Specify via input port (g)  scaleValueFracLength=14  FilterSource=Specify via dialog  dfiltObjectName=dfilt.df2tsos([1 0.3 0.4],[1 0.1 0.2])
  Out : Outport
  wires:
  Generated Filter Block/1 -> Out/1
  In/1 -> Generated Filter Block/1

== system AM_Multiple_Channels/Receiver_AM1485KHz/Asyn Demodulator/Lowpass Filter1/Lowpass Filter ==
  In : Inport
  Generated Filter Block : dsparch4/Biquad Filter  Tag=BlockMethodSubSystem  IIRFiltStruct=Direct form II  CoeffSource=Specify via dialog  BiQuadCoeffs=[1.1139495474470017e-05 2.2278990948940034e-05 1.1139495474470017e-05 1 -1.9975472496899784 0.99760587630988296;1.708449290031526e-05 3.4168985800630521e-05 1.708449290031526e-05 1 -1.99387457640288 0.99393309523238282;2.1150286544110928e-05 4.2300573088221855e-05 2.1150286544110928e-05 1 -1.9905941002634866 0.99065252281330018;2.3741131754506419e-05 4.7482263509012838e-05 2.3741131754506419e-05 1 -1.9879072271736171 0.9879655708655779;2.2148688266151217e-05 4.4297376532302434e-05 2.2148688266151217e-05 1 -1.9859774513096744 0.98603573836405833;1.4562706238119281e-05 2.9125412476238562e-05 1.4562706238119281e-05 1 -1.9849213847063547 0.98497964076591971;1.4567049256231092e-05 2.9134098512462184e-05 1.4567049256231092e-05 1 -1.9847430291087753 0.98480127993372768;1.457808673549499e-05 2.915617347098998e-05 1.457808673549499e-05 1 -1.9853349366021702 0.98539320479919512;1.4595153426943952e-05 2.9190306853887904e-05 1.4595153426943952e-05 1 -1.986839228435767 0.98689754078270897;1.4617214727563608e-05 2.9234429455127217e-05 1.4617214727563608e-05 1 -1.9891652381977778 0.98922361881148557;1.4642922502972056e-05 2.9285845005944111e-05 1.4642922502972056e-05 1 -1.9921719604380583 0.99223042929696859;8.6714112246987757e-06 1.7342822449397551e-05 8.6714112246987757e-06 1 -1.995675658652956 0.99573423034296782;6.3986527910792821e-06 1.2797305582158564e-05 6.3986527910792821e-06 1 -1.9994601364673172 0.99951881922911578;1.3142520276408514e-05 2.6285040552817028e-05 1.3142520276408514e-05 1 -1.9966044420030755 0.99666304095223146;1.8418289343954956e-05 3.6836578687909913e-05 1.8418289343954956e-05 1 -1.9930092733310447 0.99306776676450537;2.2982277427308612e-05 4.5964554854617224e-05 2.2982277427308612e-05 1 -1.9898596189140614 0.98991801990735939;2.6110938013399351e-05 5.2221876026798703e-05 2.6110938013399351e-05 1 -1.9873483912460574 0.98740671853657336;1.7614429604367743e-05 3.5228859208735487e-05 1.7614429604367743e-05 1 -1.9856280998827738 0.98568637668393688;1.4565318613601885e-05 2.9130637227203771e-05 1.4565318613601885e-05 1 -1.9848025557236171 0.98486080829563394;1.4574729484739814e-05 2.9149458969479628e-05 1.4574729484739814e-05 1 -1.9850990682844676 0.98515732955892188;1.4590372236056304e-05 2.9180744472112607e-05 1.4590372236056304e-05 1 -1.9863816706239454 0.98643996954188451;1.4611300168831942e-05 2.9222600337663884e-05 1.4611300168831942e-05 1 -1.9885136123818619 0.98857197387080598;1.4636237197718225e-05 2.9272474395436451e-05 1.4636237197718225e-05 1 -1.9913658685524318 0.99142431375310713;1.4663493412127055e-05 2.9326986824254111e-05 1.4663493412127055e-05 1 -1.9947645221736521 0.99482306712244295;0.25000264423165819 0.50000528846331638 0.25000264423165819 1 -1.9985003940838757 0.99855904867790413]  a0Flag=Warning  IC=0  ICnum=0  ICden=0  InputProcessing=Columns as channels (frame based)  denAccumFracLength=30  denProdOutputFracLength=30  secondMemoryFracLength=15  roundingMode=Floor  overflowMode=off  ScaleValues=[1.8320818000818615e-05;1;1;1;1;1;1;1;1;1;1;1;1;1;1;1;1;1;1;1;1;1;1;1;1;1]  optimizeScaleValues=off  ScaleValueMode=Specify via input port (g)  scaleValueFracLength=14  FilterSource=Specify via dialog  dfiltObjectName=dfilt.df2tsos([1 0.3 0.4],[1 0.1 0.2])
  Out : Outport
  wires:
  Generated Filter Block/1 -> Out/1
  In/1 -> Generated Filter Block/1

== system AM_Multiple_Channels/Receiver_AM639KHz/Asyn Demodulator/Lowpass Filter1/Lowpass Filter ==
  In : Inport
  Generated Filter Block : dsparch4/Biquad Filter  Tag=BlockMethodSubSystem  IIRFiltStruct=Direct form II  CoeffSource=Specify via dialog  BiQuadCoeffs=[1.1139495474470017e-05 2.2278990948940034e-05 1.1139495474470017e-05 1 -1.9975472496899784 0.99760587630988296;1.708449290031526e-05 3.4168985800630521e-05 1.708449290031526e-05 1 -1.99387457640288 0.99393309523238282;2.1150286544110928e-05 4.2300573088221855e-05 2.1150286544110928e-05 1 -1.9905941002634866 0.99065252281330018;2.3741131754506419e-05 4.7482263509012838e-05 2.3741131754506419e-05 1 -1.9879072271736171 0.9879655708655779;2.2148688266151217e-05 4.4297376532302434e-05 2.2148688266151217e-05 1 -1.9859774513096744 0.98603573836405833;1.4562706238119281e-05 2.9125412476238562e-05 1.4562706238119281e-05 1 -1.9849213847063547 0.98497964076591971;1.4567049256231092e-05 2.9134098512462184e-05 1.4567049256231092e-05 1 -1.9847430291087753 0.98480127993372768;1.457808673549499e-05 2.915617347098998e-05 1.457808673549499e-05 1 -1.9853349366021702 0.98539320479919512;1.4595153426943952e-05 2.9190306853887904e-05 1.4595153426943952e-05 1 -1.986839228435767 0.98689754078270897;1.4617214727563608e-05 2.9234429455127217e-05 1.4617214727563608e-05 1 -1.9891652381977778 0.98922361881148557;1.4642922502972056e-05 2.9285845005944111e-05 1.4642922502972056e-05 1 -1.9921719604380583 0.99223042929696859;8.6714112246987757e-06 1.7342822449397551e-05 8.6714112246987757e-06 1 -1.995675658652956 0.99573423034296782;6.3986527910792821e-06 1.2797305582158564e-05 6.3986527910792821e-06 1 -1.9994601364673172 0.99951881922911578;1.3142520276408514e-05 2.6285040552817028e-05 1.3142520276408514e-05 1 -1.9966044420030755 0.99666304095223146;1.8418289343954956e-05 3.6836578687909913e-05 1.8418289343954956e-05 1 -1.9930092733310447 0.99306776676450537;2.2982277427308612e-05 4.5964554854617224e-05 2.2982277427308612e-05 1 -1.9898596189140614 0.98991801990735939;2.6110938013399351e-05 5.2221876026798703e-05 2.6110938013399351e-05 1 -1.9873483912460574 0.98740671853657336;1.7614429604367743e-05 3.5228859208735487e-05 1.7614429604367743e-05 1 -1.9856280998827738 0.98568637668393688;1.4565318613601885e-05 2.9130637227203771e-05 1.4565318613601885e-05 1 -1.9848025557236171 0.98486080829563394;1.4574729484739814e-05 2.9149458969479628e-05 1.4574729484739814e-05 1 -1.9850990682844676 0.98515732955892188;1.4590372236056304e-05 2.9180744472112607e-05 1.4590372236056304e-05 1 -1.9863816706239454 0.98643996954188451;1.4611300168831942e-05 2.9222600337663884e-05 1.4611300168831942e-05 1 -1.9885136123818619 0.98857197387080598;1.4636237197718225e-05 2.9272474395436451e-05 1.4636237197718225e-05 1 -1.9913658685524318 0.99142431375310713;1.4663493412127055e-05 2.9326986824254111e-05 1.4663493412127055e-05 1 -1.9947645221736521 0.99482306712244295;0.25000264423165819 0.50000528846331638 0.25000264423165819 1 -1.9985003940838757 0.99855904867790413]  a0Flag=Warning  IC=0  ICnum=0  ICden=0  InputProcessing=Columns as channels (frame based)  denAccumFracLength=30  denProdOutputFracLength=30  secondMemoryFracLength=15  roundingMode=Floor  overflowMode=off  ScaleValues=[1.8320818000818615e-05;1;1;1;1;1;1;1;1;1;1;1;1;1;1;1;1;1;1;1;1;1;1;1;1;1]  optimizeScaleValues=off  ScaleValueMode=Specify via input port (g)  scaleValueFracLength=14  FilterSource=Specify via dialog  dfiltObjectName=dfilt.df2tsos([1 0.3 0.4],[1 0.1 0.2])
  Out : Outport
  wires:
  Generated Filter Block/1 -> Out/1
  In/1 -> Generated Filter Block/1

== system AM_Multiple_Channels/Receiver_AM792KHz/Asyn Demodulator/Lowpass Filter1/Lowpass Filter ==
  In : Inport
  Generated Filter Block : dsparch4/Biquad Filter  Tag=BlockMethodSubSystem  IIRFiltStruct=Direct form II  CoeffSource=Specify via dialog  BiQuadCoeffs=[1.1139495474470017e-05 2.2278990948940034e-05 1.1139495474470017e-05 1 -1.9975472496899784 0.99760587630988296;1.708449290031526e-05 3.4168985800630521e-05 1.708449290031526e-05 1 -1.99387457640288 0.99393309523238282;2.1150286544110928e-05 4.2300573088221855e-05 2.1150286544110928e-05 1 -1.9905941002634866 0.99065252281330018;2.3741131754506419e-05 4.7482263509012838e-05 2.3741131754506419e-05 1 -1.9879072271736171 0.9879655708655779;2.2148688266151217e-05 4.4297376532302434e-05 2.2148688266151217e-05 1 -1.9859774513096744 0.98603573836405833;1.4562706238119281e-05 2.9125412476238562e-05 1.4562706238119281e-05 1 -1.9849213847063547 0.98497964076591971;1.4567049256231092e-05 2.9134098512462184e-05 1.4567049256231092e-05 1 -1.9847430291087753 0.98480127993372768;1.457808673549499e-05 2.915617347098998e-05 1.457808673549499e-05 1 -1.9853349366021702 0.98539320479919512;1.4595153426943952e-05 2.9190306853887904e-05 1.4595153426943952e-05 1 -1.986839228435767 0.98689754078270897;1.4617214727563608e-05 2.9234429455127217e-05 1.4617214727563608e-05 1 -1.9891652381977778 0.98922361881148557;1.4642922502972056e-05 2.9285845005944111e-05 1.4642922502972056e-05 1 -1.9921719604380583 0.99223042929696859;8.6714112246987757e-06 1.7342822449397551e-05 8.6714112246987757e-06 1 -1.995675658652956 0.99573423034296782;6.3986527910792821e-06 1.2797305582158564e-05 6.3986527910792821e-06 1 -1.9994601364673172 0.99951881922911578;1.3142520276408514e-05 2.6285040552817028e-05 1.3142520276408514e-05 1 -1.9966044420030755 0.99666304095223146;1.8418289343954956e-05 3.6836578687909913e-05 1.8418289343954956e-05 1 -1.9930092733310447 0.99306776676450537;2.2982277427308612e-05 4.5964554854617224e-05 2.2982277427308612e-05 1 -1.9898596189140614 0.98991801990735939;2.6110938013399351e-05 5.2221876026798703e-05 2.6110938013399351e-05 1 -1.9873483912460574 0.98740671853657336;1.7614429604367743e-05 3.5228859208735487e-05 1.7614429604367743e-05 1 -1.9856280998827738 0.98568637668393688;1.4565318613601885e-05 2.9130637227203771e-05 1.4565318613601885e-05 1 -1.9848025557236171 0.98486080829563394;1.4574729484739814e-05 2.9149458969479628e-05 1.4574729484739814e-05 1 -1.9850990682844676 0.98515732955892188;1.4590372236056304e-05 2.9180744472112607e-05 1.4590372236056304e-05 1 -1.9863816706239454 0.98643996954188451;1.4611300168831942e-05 2.9222600337663884e-05 1.4611300168831942e-05 1 -1.9885136123818619 0.98857197387080598;1.4636237197718225e-05 2.9272474395436451e-05 1.4636237197718225e-05 1 -1.9913658685524318 0.99142431375310713;1.4663493412127055e-05 2.9326986824254111e-05 1.4663493412127055e-05 1 -1.9947645221736521 0.99482306712244295;0.25000264423165819 0.50000528846331638 0.25000264423165819 1 -1.9985003940838757 0.99855904867790413]  a0Flag=Warning  IC=0  ICnum=0  ICden=0  InputProcessing=Columns as channels (frame based)  denAccumFracLength=30  denProdOutputFracLength=30  secondMemoryFracLength=15  roundingMode=Floor  overflowMode=off  ScaleValues=[1.8320818000818615e-05;1;1;1;1;1;1;1;1;1;1;1;1;1;1;1;1;1;1;1;1;1;1;1;1;1]  optimizeScaleValues=off  ScaleValueMode=Specify via input port (g)  scaleValueFracLength=14  FilterSource=Specify via dialog  dfiltObjectName=dfilt.df2tsos([1 0.3 0.4],[1 0.1 0.2])
  Out : Outport
  wires:
  Generated Filter Block/1 -> Out/1
  In/1 -> Generated Filter Block/1
